simulink model "Truth_Table"  (R2024a)
settings: Solver=VariableStepAuto  StartTime=0.0  StopTime=10.0  RelTol=1e-3
settings Model: Creator=VICTUS  LastModifiedBy=VICTUS

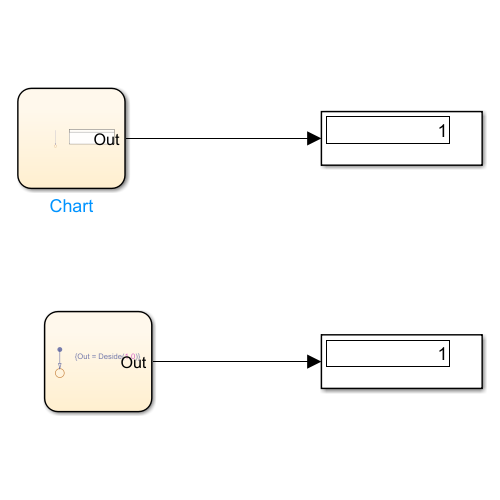
[thumbnail: Simulink's stored preview of the top-level diagram]
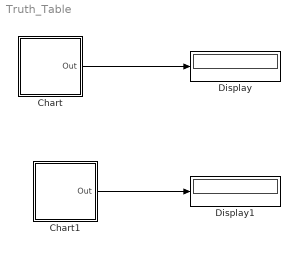
== system Truth_Table ==
  Chart : Stateflow chart  TreatAsAtomicUnit=on
  Chart1 : Stateflow chart  TreatAsAtomicUnit=on
  Display : Display
  Display1 : Display
  wires:
  Chart/1(Out) -> Display/1
  Chart1/1(Out) -> Display1/1

== stateflow chart Truth_Table/Chart1 ==
  (default) -> (junction 9) : {Out = Deside(1,0)}
  data: Out output double

== matlab function Truth_Table/Chart ==
  data: IN1 function_input double; IN2 function_input double; Out function_output double; Out output
function Out = Deside(IN1,IN2)

aVarTruthTableCondition_1 = false;
aVarTruthTableCondition_2 = false;


% Condition #1
aVarTruthTableCondition_1 = logical(IN2);

% Condition #2
aVarTruthTableCondition_2 = logical(IN1);

if (~aVarTruthTableCondition_1 && aVarTruthTableCondition_2)
    aFcnTruthTableAction_1();
elseif (aVarTruthTableCondition_1 && ~aVarTruthTableCondition_2)
    aFcnTruthTableAction_2();
elseif (~aVarTruthTableCondition_1 && ~aVarTruthTableCondition_2)
    aFcnTruthTableAction_3();
else % Default
    aFcnTruthTableAction_4();
end

function aFcnTruthTableAction_1()



Out= 1;

function aFcnTruthTableAction_2()



Out= 2;

function aFcnTruthTableAction_3()



Out= 3;

function aFcnTruthTableAction_4()



Out= 4;
